simulink model "kopter_se_zavazim_LQR"  (R2024b)
settings: Solver=FixedStepAuto  StartTime=0.0  StopTime=30  FixedStep=0.01  RelTol=1e-3
values from neighbouring files (symbols this model uses):
  b_moment = 5.4e-6    (= 5.4e-06)    [parametry_kopter_se_zavazim.m]
  d = 1    [parametry_kopter_se_zavazim.m]
  g = 9.81    [parametry_kopter_se_zavazim.m]
  Ip = m*d^2    (= 1)    [parametry_kopter_se_zavazim.m]
  Ixx = 0.0222    [parametry_kopter_se_zavazim.m]
  Iyy = 0.0222    [parametry_kopter_se_zavazim.m]
  Izz = 0.0429    [parametry_kopter_se_zavazim.m]
  k_thrust = 2.3e-3    (= 0.0023)    [parametry_kopter_se_zavazim.m]
  ki_lqr = K_ex_lqr(:, 17:20)    [odvozeni_stavova_regulace_OTHER_ANGLES.m]
  kimot_lqr = Kmot_ex_lqr(:, 17:20)    [odvozeni_stavova_regulace_OTHER_ANGLES.m]
  kp_lqr = K_ex_lqr(:, 1:16)    [odvozeni_stavova_regulace_OTHER_ANGLES.m]
  kpmot_lqr = Kmot_ex_lqr(:, 1:16)    [odvozeni_stavova_regulace_OTHER_ANGLES.m]
  l = 0.2051    [parametry_kopter_se_zavazim.m]
  L_observer = place(Ac', Cc', poles_obs)'    [odvozeni_stavova_regulace_OTHER_ANGLES.m]
  M = 2    [parametry_kopter_se_zavazim.m]
  m = 1    [parametry_kopter_se_zavazim.m]
  Us_p = [(M+m)*g; 0; 0; 0]    [parametry_kopter_se_zavazim.m]
  Xinit_ss = [Xinit_matrix; [0 0 0 0 0 0 0 0]']    [parametry_kopter_se_zavazim.m]
  Xs_p = [0;0;0; 0;0;0; 0;0; 0;0;0; 0;0;0; 0;0]    [parametry_kopter_se_zavazim.m]
undefined symbols (not defined in the file or in its folder): L
libraries: simulink_extras x10
(part 1 of 3)
settings Model: Creator=Admin  LastModifiedBy=Admin

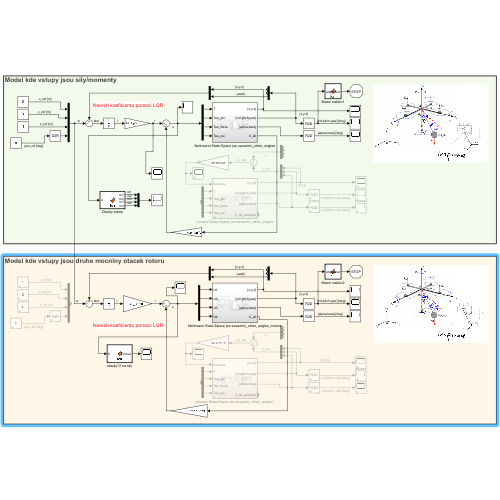
[thumbnail: Simulink's stored preview of the top-level diagram]
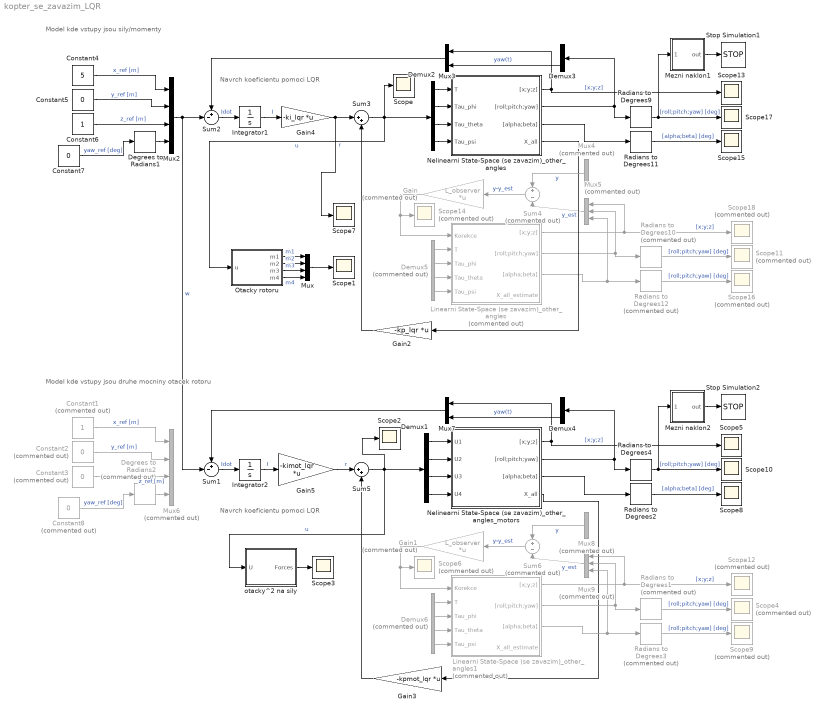
== system kopter_se_zavazim_LQR ==
  note: Navrch koeficientu pomoci LQR
  note: Model kde vstupy jsou sily/momenty
  note: Model kde vstupy jsou druhe mocniny otacek rotoru
  note: Navrch koeficientu pomoci LQR
  Constant1 : Constant  Commented=on
  Constant2 : Constant  Commented=on  Value=0
  Constant3 : Constant  Commented=on  Value=0
  Constant4 : Constant  Value=5
  Constant5 : Constant  Value=0
  Constant6 : Constant
  Constant7 : Constant  Value=0
  Constant8 : Constant  Commented=on  Value=0
  Degrees to Radians1 : simulink_extras/Transformations/Degrees to Radians
  Degrees to Radians2 : simulink_extras/Transformations/Degrees to Radians  Commented=on
  Demux1 : Demux
  Demux2 : Demux
  Demux3 : Demux  Outputs=3
  Demux4 : Demux  Outputs=3
  Demux5 : Demux  Commented=on
  Demux6 : Demux  Commented=on
  Gain : Gain  Commented=on  Gain=L_observer  Multiplication=Matrix(K*u)
  Gain1 : Gain  Commented=on  Gain=L_observer  Multiplication=Matrix(K*u)
  Gain2 : Gain  Gain=-kp_lqr  Multiplication=Matrix(K*u)
  Gain3 : Gain  Gain=-kpmot_lqr  Multiplication=Matrix(K*u)
  Gain4 : Gain  Gain=-ki_lqr  Multiplication=Matrix(K*u)
  Gain5 : Gain  Gain=-kimot_lqr  Multiplication=Matrix(K*u)
  Integrator1 : Integrator
  Integrator2 : Integrator
  Linearni State-Space (se zavazim)_other_angles : Subsystem  Commented=on
  Linearni State-Space (se zavazim)_other_angles1 : Subsystem  Commented=on
  Mezni naklon1 : MATLAB Function  TreatAsAtomicUnit=on
  Mezni naklon2 : MATLAB Function  TreatAsAtomicUnit=on
  Mux : Mux
  Mux2 : Mux
  Mux3 : Mux  Inputs=2
  Mux{4..5,8..9} (4 alike) : Mux  Commented=on  Inputs=3
  Mux6 : Mux  Commented=on
  Mux7 : Mux  Inputs=2
  Nelinearni State-Space (se zavazim)_other_angles : Subsystem
  Nelinearni State-Space (se zavazim)_other_angles_motors : Subsystem
  Otacky rotoru : MATLAB Function  TreatAsAtomicUnit=on
  Radians to Degrees{1,3,10,12} (4 alike) : simulink_extras/Transformations/Radians to Degrees  Commented=on
  Radians to Degrees{2,4,9,11} (4 alike) : simulink_extras/Transformations/Radians to Degrees
  Scope{,1..3,5,7..8,10,13,15,17} (11 alike) : Scope
  Scope{4,6,9,11..12,14,16,18} (8 alike) : Scope  Commented=on
  Stop Simulation1 : Stop
  Stop Simulation2 : Stop
  Sum1 : Sum  Inputs=+-|
  Sum2 : Sum  Inputs=+-|
  Sum3 : Sum  Inputs=|++
  Sum4 : Sum  Commented=on  Inputs=+|-
  Sum5 : Sum  Inputs=|++
  Sum6 : Sum  Commented=on  Inputs=+|-
  otacky^2 na sily : MATLAB Function  TreatAsAtomicUnit=on
  wires:
  Linearni State-Space (se zavazim)_other_angles/1("[x;y;z]") -> Mux5/1, Scope18/1  "[x;y;z]"
  Demux5/3 -> Linearni State-Space (se zavazim)_other_angles/4(Tau_theta)
  Demux5/2 -> Linearni State-Space (se zavazim)_other_angles/3(Tau_phi)
  Nelinearni State-Space (se zavazim)_other_angles/3("[alpha;beta]") -> Radians to Degrees11/1
  Linearni State-Space (se zavazim)_other_angles/3("[alpha;beta]") -> Mux5/3, Radians to Degrees12/1
  Radians to Degrees10/1 -> Scope11/1  "[roll;pitch;yaw] [deg]"
  Linearni State-Space (se zavazim)_other_angles/2("[roll;pitch;yaw]") -> Mux5/2, Radians to Degrees10/1
  Radians to Degrees12/1 -> Scope16/1  "[roll;pitch;yaw] [deg]"
  Demux5/1 -> Linearni State-Space (se zavazim)_other_angles/2(T)
  Demux5/4 -> Linearni State-Space (se zavazim)_other_angles/5(Tau_psi)
  Radians to Degrees9/1 -> Scope17/1, Mezni naklon1/1(angles)  "[roll;pitch;yaw] [deg]"
  Radians to Degrees11/1 -> Scope15/1  "[alpha;beta] [deg]"
  Demux2/3 -> Nelinearni State-Space (se zavazim)_other_angles/3(Tau_theta)
  Demux2/2 -> Nelinearni State-Space (se zavazim)_other_angles/2(Tau_phi)
  Constant5/1 -> Mux2/2  "y_ref [m]"
  Constant7/1 -> Degrees to Radians1/1  "yaw_ref [deg]"
  Constant6/1 -> Mux2/3  "z_ref [m]"
  Gain2/1 -> Sum3/2
  Sum3/1 -> Otacky rotoru/1(u), Scope/1, Demux2/1  "u"
  Mux3/1 -> Sum2/1
  Demux2/4 -> Nelinearni State-Space (se zavazim)_other_angles/4(Tau_psi)
  Sum2/1 -> Integrator1/1  "Idot"
  Gain4/1 -> Scope7/1, Sum3/1  "r"
  Demux2/1 -> Nelinearni State-Space (se zavazim)_other_angles/1(T)
  Integrator1/1 -> Gain4/1  "I"
  Degrees to Radians1/1 -> Mux2/4
  Constant4/1 -> Mux2/1  "x_ref [m]"
  Demux3/3 -> Mux3/2  "yaw(t)"
  Nelinearni State-Space (se zavazim)_other_angles/1("[x;y;z]") -> Scope13/1, Mux3/1  "[x;y;z]"
  Nelinearni State-Space (se zavazim)_other_angles/2("[roll;pitch;yaw]") -> Radians to Degrees9/1, Demux3/1
  Mezni naklon1/1(out) -> Stop Simulation1/1
  Nelinearni State-Space (se zavazim)_other_angles/4(X_all) -> Gain2/1
  Gain/1 -> Scope14/1, Linearni State-Space (se zavazim)_other_angles/1(Korekce)
  Sum4/1 -> Gain/1  "y-y_est"
  Mux4/1 -> Sum4/1  "y"
  Mux5/1 -> Sum4/2  "y_est"
  Otacky rotoru/1(m1) -> Mux/1  "m1"
  Otacky rotoru/2(m2) -> Mux/2  "m2"
  Otacky rotoru/3(m3) -> Mux/3  "m3"
  Otacky rotoru/4(m4) -> Mux/4  "m4"
  Mux/1 -> Scope1/1
  Radians to Degrees4/1 -> Scope10/1, Mezni naklon2/1(angles)  "[roll;pitch;yaw] [deg]"
  Demux6/2 -> Linearni State-Space (se zavazim)_other_angles1/3(Tau_phi)
  Integrator2/1 -> Gain5/1  "I"
  Radians to Degrees2/1 -> Scope8/1  "[alpha;beta] [deg]"
  Gain1/1 -> Scope6/1, Linearni State-Space (se zavazim)_other_angles1/1(Korekce)
  Nelinearni State-Space (se zavazim)_other_angles_motors/4(X_all) -> Gain3/1
  Nelinearni State-Space (se zavazim)_other_angles_motors/2("[roll;pitch;yaw]") -> Radians to Degrees4/1, Demux4/1
  Sum5/1 -> otacky^2 na sily/1(U), Scope2/1, Demux1/1  "u"
  Sum1/1 -> Integrator2/1  "Idot"
  Demux1/2 -> Nelinearni State-Space (se zavazim)_other_angles_motors/2(U2)
  Linearni State-Space (se zavazim)_other_angles1/3("[alpha;beta]") -> Mux9/3, Radians to Degrees3/1
  Degrees to Radians2/1 -> Mux6/4
  Demux6/3 -> Linearni State-Space (se zavazim)_other_angles1/4(Tau_theta)
  Constant2/1 -> Mux6/2  "y_ref [m]"
  Demux4/3 -> Mux7/2  "yaw(t)"
  Demux1/3 -> Nelinearni State-Space (se zavazim)_other_angles_motors/3(U3)
  Constant3/1 -> Mux6/3  "z_ref [m]"
  Mux2/1 -> Sum2/2, Sum1/2  "w"
  Nelinearni State-Space (se zavazim)_other_angles_motors/3("[alpha;beta]") -> Radians to Degrees2/1
  Mux9/1 -> Sum6/2  "y_est"
  Nelinearni State-Space (se zavazim)_other_angles_motors/1("[x;y;z]") -> Scope5/1, Mux7/1  "[x;y;z]"
  Sum6/1 -> Gain1/1  "y-y_est"
  Demux1/1 -> Nelinearni State-Space (se zavazim)_other_angles_motors/1(U1)
  Linearni State-Space (se zavazim)_other_angles1/1("[x;y;z]") -> Mux9/1, Scope12/1  "[x;y;z]"
  Mux7/1 -> Sum1/1
  Mezni naklon2/1(out) -> Stop Simulation2/1
  Radians to Degrees1/1 -> Scope4/1  "[roll;pitch;yaw] [deg]"
  Mux8/1 -> Sum6/1  "y"
  Gain3/1 -> Sum5/2
  Radians to Degrees3/1 -> Scope9/1  "[roll;pitch;yaw] [deg]"
  Gain5/1 -> Sum5/1  "r"
  Linearni State-Space (se zavazim)_other_angles1/2("[roll;pitch;yaw]") -> Mux9/2, Radians to Degrees1/1
  Demux6/1 -> Linearni State-Space (se zavazim)_other_angles1/2(T)
  Demux6/4 -> Linearni State-Space (se zavazim)_other_angles1/5(Tau_psi)
  Demux1/4 -> Nelinearni State-Space (se zavazim)_other_angles_motors/4(U4)
  Constant8/1 -> Degrees to Radians2/1  "yaw_ref [deg]"
  Constant1/1 -> Mux6/1  "x_ref [m]"
  otacky^2 na sily/1(Forces) -> Scope3/1

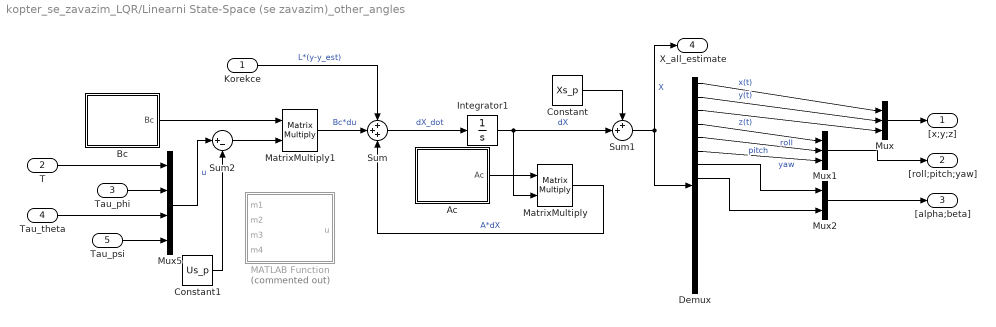
== system kopter_se_zavazim_LQR/Linearni State-Space (se zavazim)_other_angles ==
  Korekce : Inport
  T : Inport  Port=2
  Tau_phi : Inport  Port=3
  Tau_theta : Inport  Port=4
  Tau_psi : Inport  Port=5
  Ac : MATLAB Function  TreatAsAtomicUnit=on
  Bc : MATLAB Function  TreatAsAtomicUnit=on
  Constant : Constant  Value=Xs_p
  Constant1 : Constant  Value=Us_p
  Demux : Demux  Outputs=16
  Integrator1 : Integrator  InitialCondition=Xinit_ss
  MATLAB Function : MATLAB Function  Commented=on  TreatAsAtomicUnit=on
  MatrixMultiply : Product  Multiplication=Matrix(*)
  MatrixMultiply1 : Product  Multiplication=Matrix(*)
  Mux : Mux  Inputs=3
  Mux1 : Mux  Inputs=3
  Mux2 : Mux  Inputs=2
  Mux5 : Mux
  Sum : Sum  Inputs=+++
  Sum1 : Sum  Inputs=++|
  Sum2 : Sum  Inputs=|+-
  "[x;y;z]" : Outport
  "[roll;pitch;yaw]" : Outport  Port=2
  "[alpha;beta]" : Outport  Port=3
  X_all_estimate : Outport  Port=4
  wires:
  Mux5/1 -> Sum2/1  "u"
  Ac/1(Ac) -> MatrixMultiply/1
  Integrator1/1 -> Sum1/2, MatrixMultiply/2  "dX"
  Demux/1 -> Mux/1  "x(t)"
  Demux/2 -> Mux/2  "y(t)"
  Demux/3 -> Mux/3  "z(t)"
  Mux/1 -> "[x;y;z]"/1
  Demux/4 -> Mux1/1  "roll"
  Demux/5 -> Mux1/2  "pitch"
  Demux/6 -> Mux1/3  "yaw"
  Mux1/1 -> "[roll;pitch;yaw]"/1
  Sum/1 -> Integrator1/1  "dX_dot"
  MatrixMultiply1/1 -> Sum/2  "Bc*du"
  MatrixMultiply/1 -> Sum/3  "A*dX"
  Bc/1(Bc) -> MatrixMultiply1/1
  Sum1/1 -> Demux/1, X_all_estimate/1  "X"
  Constant/1 -> Sum1/1
  Constant1/1 -> Sum2/2
  Sum2/1 -> MatrixMultiply1/2
  Mux2/1 -> "[alpha;beta]"/1
  Demux/7 -> Mux2/1
  Demux/8 -> Mux2/2
  Tau_psi/1 -> Mux5/4
  T/1 -> Mux5/1
  Tau_theta/1 -> Mux5/3
  Tau_phi/1 -> Mux5/2
  Korekce/1 -> Sum/1  "L*(y-y_est)"

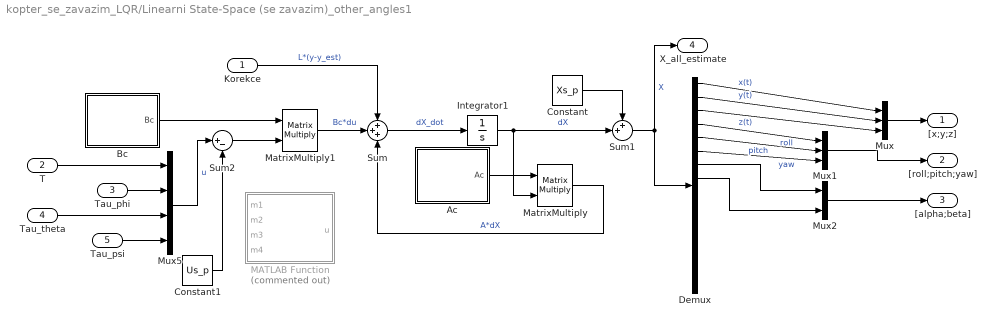
== system kopter_se_zavazim_LQR/Linearni State-Space (se zavazim)_other_angles1 ==
  Korekce : Inport
  T : Inport  Port=2
  Tau_phi : Inport  Port=3
  Tau_theta : Inport  Port=4
  Tau_psi : Inport  Port=5
  Ac : MATLAB Function  TreatAsAtomicUnit=on
  Bc : MATLAB Function  TreatAsAtomicUnit=on
  Constant : Constant  Value=Xs_p
  Constant1 : Constant  Value=Us_p
  Demux : Demux  Outputs=16
  Integrator1 : Integrator  InitialCondition=Xinit_ss
  MATLAB Function : MATLAB Function  Commented=on  TreatAsAtomicUnit=on
  MatrixMultiply : Product  Multiplication=Matrix(*)
  MatrixMultiply1 : Product  Multiplication=Matrix(*)
  Mux : Mux  Inputs=3
  Mux1 : Mux  Inputs=3
  Mux2 : Mux  Inputs=2
  Mux5 : Mux
  Sum : Sum  Inputs=+++
  Sum1 : Sum  Inputs=++|
  Sum2 : Sum  Inputs=|+-
  "[x;y;z]" : Outport
  "[roll;pitch;yaw]" : Outport  Port=2
  "[alpha;beta]" : Outport  Port=3
  X_all_estimate : Outport  Port=4
  wires:
  Mux5/1 -> Sum2/1  "u"
  Ac/1(Ac) -> MatrixMultiply/1
  Integrator1/1 -> Sum1/2, MatrixMultiply/2  "dX"
  Demux/1 -> Mux/1  "x(t)"
  Demux/2 -> Mux/2  "y(t)"
  Demux/3 -> Mux/3  "z(t)"
  Mux/1 -> "[x;y;z]"/1
  Demux/4 -> Mux1/1  "roll"
  Demux/5 -> Mux1/2  "pitch"
  Demux/6 -> Mux1/3  "yaw"
  Mux1/1 -> "[roll;pitch;yaw]"/1
  Sum/1 -> Integrator1/1  "dX_dot"
  MatrixMultiply1/1 -> Sum/2  "Bc*du"
  MatrixMultiply/1 -> Sum/3  "A*dX"
  Bc/1(Bc) -> MatrixMultiply1/1
  Sum1/1 -> Demux/1, X_all_estimate/1  "X"
  Constant/1 -> Sum1/1
  Constant1/1 -> Sum2/2
  Sum2/1 -> MatrixMultiply1/2
  Mux2/1 -> "[alpha;beta]"/1
  Demux/7 -> Mux2/1
  Demux/8 -> Mux2/2
  Tau_psi/1 -> Mux5/4
  T/1 -> Mux5/1
  Tau_theta/1 -> Mux5/3
  Tau_phi/1 -> Mux5/2
  Korekce/1 -> Sum/1  "L*(y-y_est)"

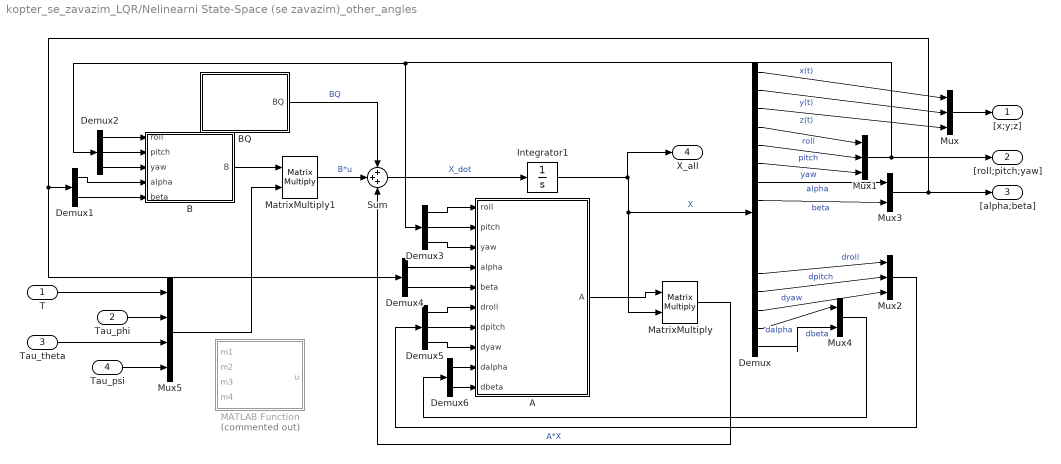
== system kopter_se_zavazim_LQR/Nelinearni State-Space (se zavazim)_other_angles ==
  T : Inport
  Tau_phi : Inport  Port=2
  Tau_theta : Inport  Port=3
  Tau_psi : Inport  Port=4
  A : MATLAB Function  TreatAsAtomicUnit=on
  B : MATLAB Function  TreatAsAtomicUnit=on
  BQ : MATLAB Function  TreatAsAtomicUnit=on
  Demux : Demux  Outputs=16
  Demux1 : Demux  Outputs=2
  Demux2 : Demux  Outputs=3
  Demux3 : Demux  Outputs=3
  Demux4 : Demux  Outputs=2
  Demux5 : Demux  Outputs=3
  Demux6 : Demux  Outputs=2
  Integrator1 : Integrator  InitialCondition=Xinit_ss
  MATLAB Function : MATLAB Function  Commented=on  TreatAsAtomicUnit=on
  MatrixMultiply : Product  Multiplication=Matrix(*)
  MatrixMultiply1 : Product  Multiplication=Matrix(*)
  Mux : Mux  Inputs=3
  Mux1 : Mux  Inputs=3
  Mux2 : Mux  Inputs=3
  Mux3 : Mux  Inputs=2
  Mux4 : Mux  Inputs=2
  Mux5 : Mux
  Sum : Sum  Inputs=+++
  "[x;y;z]" : Outport
  "[roll;pitch;yaw]" : Outport  Port=2
  "[alpha;beta]" : Outport  Port=3
  X_all : Outport  Port=4
  wires:
  A/1(A) -> MatrixMultiply/1
  Integrator1/1 -> X_all/1, MatrixMultiply/2, Demux/1  "X"
  Demux/1 -> Mux/1  "x(t)"
  Demux/2 -> Mux/2  "y(t)"
  Demux/3 -> Mux/3  "z(t)"
  Mux/1 -> "[x;y;z]"/1
  Demux/4 -> Mux1/1  "roll"
  Demux/5 -> Mux1/2  "pitch"
  Demux/6 -> Mux1/3  "yaw"
  Mux1/1 -> Demux2/1, Demux3/1, "[roll;pitch;yaw]"/1
  Demux/12 -> Mux2/1  "droll"
  Demux/13 -> Mux2/2  "dpitch"
  Demux/14 -> Mux2/3  "dyaw"
  Demux2/1 -> B/1(roll)
  Demux2/2 -> B/2(pitch)
  Demux2/3 -> B/3(yaw)
  Demux3/2 -> A/2(pitch)
  Demux3/1 -> A/1(roll)
  Demux3/3 -> A/3(yaw)
  Demux5/2 -> A/7(dpitch)
  Demux5/1 -> A/6(droll)
  Demux5/3 -> A/8(dyaw)
  Sum/1 -> Integrator1/1  "X_dot"
  BQ/1(BQ) -> Sum/1  "BQ"
  MatrixMultiply1/1 -> Sum/2  "B*u"
  B/1(B) -> MatrixMultiply1/1
  MatrixMultiply/1 -> Sum/3  "A*X"
  Mux2/1 -> Demux5/1
  Demux/7 -> Mux3/1  "alpha"
  Demux/8 -> Mux3/2  "beta"
  Mux3/1 -> Demux4/1, Demux1/1, "[alpha;beta]"/1
  Demux1/2 -> B/5(beta)
  Demux1/1 -> B/4(alpha)
  Demux4/2 -> A/5(beta)
  Demux4/1 -> A/4(alpha)
  Demux/15 -> Mux4/1  "dalpha"
  Demux/16 -> Mux4/2  "dbeta"
  Demux6/1 -> A/9(dalpha)
  Demux6/2 -> A/10(dbeta)
  Mux4/1 -> Demux6/1
  Tau_theta/1 -> Mux5/3
  Tau_psi/1 -> Mux5/4
  Tau_phi/1 -> Mux5/2
  Mux5/1 -> MatrixMultiply1/2
  T/1 -> Mux5/1

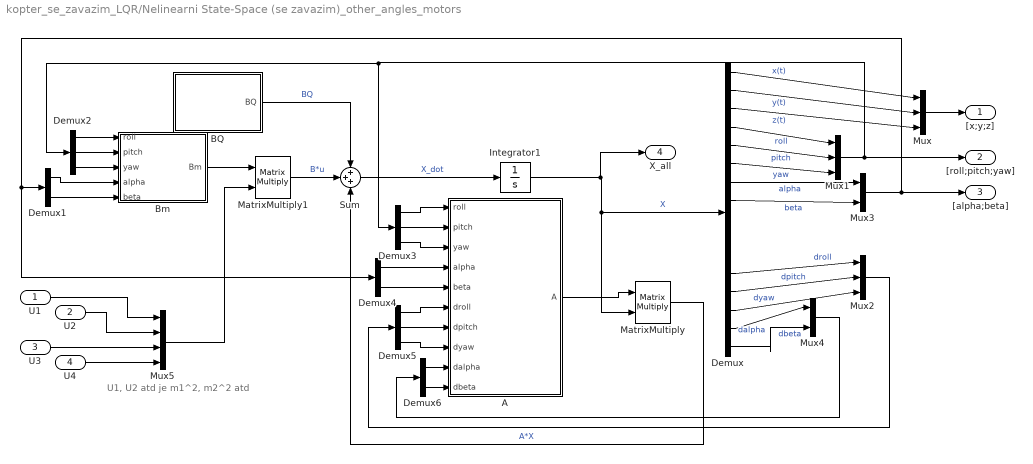
== system kopter_se_zavazim_LQR/Nelinearni State-Space (se zavazim)_other_angles_motors ==
  note: U1, U2 atd je m1^2, m2^2 atd
  U1 : Inport
  U2 : Inport  Port=2
  U3 : Inport  Port=3
  U4 : Inport  Port=4
  A : MATLAB Function  TreatAsAtomicUnit=on
  BQ : MATLAB Function  TreatAsAtomicUnit=on
  Bm : MATLAB Function  TreatAsAtomicUnit=on
  Demux : Demux  Outputs=16
  Demux1 : Demux  Outputs=2
  Demux2 : Demux  Outputs=3
  Demux3 : Demux  Outputs=3
  Demux4 : Demux  Outputs=2
  Demux5 : Demux  Outputs=3
  Demux6 : Demux  Outputs=2
  Integrator1 : Integrator  InitialCondition=Xinit_ss
  MatrixMultiply : Product  Multiplication=Matrix(*)
  MatrixMultiply1 : Product  Multiplication=Matrix(*)
  Mux : Mux  Inputs=3
  Mux1 : Mux  Inputs=3
  Mux2 : Mux  Inputs=3
  Mux3 : Mux  Inputs=2
  Mux4 : Mux  Inputs=2
  Mux5 : Mux
  Sum : Sum  Inputs=+++
  "[x;y;z]" : Outport
  "[roll;pitch;yaw]" : Outport  Port=2
  "[alpha;beta]" : Outport  Port=3
  X_all : Outport  Port=4
  wires:
  A/1(A) -> MatrixMultiply/1
  Integrator1/1 -> X_all/1, MatrixMultiply/2, Demux/1  "X"
  Demux/1 -> Mux/1  "x(t)"
  Demux/2 -> Mux/2  "y(t)"
  Demux/3 -> Mux/3  "z(t)"
  Mux/1 -> "[x;y;z]"/1
  Demux/4 -> Mux1/1  "roll"
  Demux/5 -> Mux1/2  "pitch"
  Demux/6 -> Mux1/3  "yaw"
  Mux1/1 -> Demux2/1, Demux3/1, "[roll;pitch;yaw]"/1
  Demux/12 -> Mux2/1  "droll"
  Demux/13 -> Mux2/2  "dpitch"
  Demux/14 -> Mux2/3  "dyaw"
  Demux2/1 -> Bm/1(roll)
  Demux2/2 -> Bm/2(pitch)
  Demux2/3 -> Bm/3(yaw)
  Demux3/2 -> A/2(pitch)
  Demux3/1 -> A/1(roll)
  Demux3/3 -> A/3(yaw)
  Demux5/2 -> A/7(dpitch)
  Demux5/1 -> A/6(droll)
  Demux5/3 -> A/8(dyaw)
  Sum/1 -> Integrator1/1  "X_dot"
  BQ/1(BQ) -> Sum/1  "BQ"
  MatrixMultiply1/1 -> Sum/2  "B*u"
  Bm/1(Bm) -> MatrixMultiply1/1
  MatrixMultiply/1 -> Sum/3  "A*X"
  Mux2/1 -> Demux5/1
  Demux/7 -> Mux3/1  "alpha"
  Demux/8 -> Mux3/2  "beta"
  Mux3/1 -> Demux4/1, Demux1/1, "[alpha;beta]"/1
  Demux1/2 -> Bm/5(beta)
  Demux1/1 -> Bm/4(alpha)
  Demux4/2 -> A/5(beta)
  Demux4/1 -> A/4(alpha)
  Demux/15 -> Mux4/1  "dalpha"
  Demux/16 -> Mux4/2  "dbeta"
  Demux6/1 -> A/9(dalpha)
  Demux6/2 -> A/10(dbeta)
  Mux4/1 -> Demux6/1
  Mux5/1 -> MatrixMultiply1/2
  U4/1 -> Mux5/4
  U3/1 -> Mux5/3
  U2/1 -> Mux5/2
  U1/1 -> Mux5/1

== matlab function kopter_se_zavazim_LQR/Linearni State-Space (se zavazim)_other_angles1/MATLAB Function ==
  data: u output; m1 input; m2 input; m3 input; m4 input; k_thrust parameter; b_moment parameter; L parameter
function u = fcn(m1, m2, m3, m4, k_thrust, b_moment, L)

Thrust = k_thrust*(m1^2 + m2^2 + m3^2 + m4^2);
Tau_roll = L*k_thrust*(m1^2 + m4^2 - m2^2 - m3^2);
Tau_pitch = L*k_thrust*(m4^2 + m3^2 - m1^2 - m2^2);
Tau_yaw = b_moment*(m1^2 + m3^2 - m2^2 - m4^2);

u = [Thrust; Tau_roll; Tau_pitch; Tau_yaw];

== matlab function kopter_se_zavazim_LQR/Mezni naklon2 ==
  data: angles input; out output
function out = fcn(angles)

if all(angles<=85) && all(angles>=-85)
    out = 0;
else
    out = 1;
end

== matlab function kopter_se_zavazim_LQR/Nelinearni State-Space (se zavazim)_other_angles_motors/A ==
  data: roll input; A output; pitch input; yaw input; alpha input; beta input; droll input; dpitch input; dyaw input; dalpha input; dbeta input; Ixx parameter; Iyy parameter; Izz parameter; M parameter; Ip parameter; d parameter; m parameter
function A = fcn(roll, pitch, yaw, alpha, beta, droll, dpitch, dyaw, dalpha, dbeta, Ixx, Iyy, Izz, M, Ip, d, m)
% Matice dynamiky A

phi_t = roll;
theta_t = pitch;
psi_t = yaw;

alpha_t = alpha;
beta_t = beta;

phi_dot_t = droll;
theta_dot_t = dpitch;
psi_dot_t = dyaw;

alpha_dot_t = dalpha;
beta_dot_t = dbeta;

A = [ 
0, 0, 0, 0, 0, 0, 0, 0, 1, 0, 0,                                                                                                                                                                                                                                                                                                                                                                                                                                                                                                           0,                                                                                                                                                                                                                                                                                                                                                                                                                                                                                                                                                                                                                                                                                                                              0,                                                                                                                                                                                            0,                                                          0,                                                  0;
0, 0, 0, 0, 0, 0, 0, 0, 0, 1, 0,                                                                                                                                                                                                                                                                                                                                                                                                                                                                                                           0,                                                                                                                                                                                                                                                                                                                                                                                                                                                                                                                                                                                                                                                                                                                              0,                                                                                                                                                                                            0,                                                          0,                                                  0;
0, 0, 0, 0, 0, 0, 0, 0, 0, 0, 1,                                                                                                                                                                                                                                                                                                                                                                                                                                                                                                           0,                                                                                                                                                                                                                                                                                                                                                                                                                                                                                                                                                                                                                                                                                                                              0,                                                                                                                                                                                            0,                                                          0,                                                  0;
0, 0, 0, 0, 0, 0, 0, 0, 0, 0, 0,                                                                                                                                                                                                                                                                                                                                                                                                                                                                                                           1,                                                                                                                                                                                                                                                                                                                                                                                                                                                                                                                                                                                                                                                                                                                              0,                                                                                                                                                                                            0,                                                          0,                                                  0;
0, 0, 0, 0, 0, 0, 0, 0, 0, 0, 0,                                                                                                                                                                                                                                                                                                                                                                                                                                                                                                           0,                                                                                                                                                                                                                                                                                                                                                                                                                                                                                                                                                                                                                                                                                                                              1,                                                                                                                                                                                            0,                                                          0,                                                  0;
0, 0, 0, 0, 0, 0, 0, 0, 0, 0, 0,                                                                                                                                                                                                                                                                                                                                                                                                                                                                                                           0,                                                                                                                                                                                                                                                                                                                                                                                                                                                                                                                                                                                                                                                                                                                              0,                                                                                                                                                                                            1,                                                          0,                                                  0;
0, 0, 0, 0, 0, 0, 0, 0, 0, 0, 0,                                                                                                                                                                                                                                                                                                                                                                                                                                                                                                           0,                                                                                                                                                                                                                                                                                                                                                                                                                                                                                                                                                                                                                                                                                                                              0,                                                                                                                                                                                            0,                                                          1,                                                  0;
0, 0, 0, 0, 0, 0, 0, 0, 0, 0, 0,                                                                                                                                                                                                                                                                                                                                                                                                                                                                                                           0,                                                                                                                                                                                                                                                                                                                                                                                                                                                                                                                                                                                                                                                                                                                              0,                                                                                                                                                                                            0,                                                          0,                                                  1;
0, 0, 0, 0, 0, 0, 0, 0, 0, 0, 0,                                                                                                                                                                                                                                                                                                                                                                                                                                                                                                           0,                                                                                                                                                                                                                                                                                                                                                                                                                                                                                                                                                                                                                                                                                                                              0,                                                                                                                                                                                            0,       (alpha_dot_t*d*m*cos(beta_t)^3*sin(alpha_t))/(M + m),  (beta_dot_t*d*m*cos(beta_t)*sin(alpha_t))/(M + m);
0, 0, 0, 0, 0, 0, 0, 0, 0, 0, 0,                                                                                                                                                                                                                                                                                                                                                                                                                                                                                                           0,                                                                                                                                                                                                                                                                                                                                                                                                                                                                                                                                                                                                                                                                                                                              0,                                                                                                                                                                                            0, -(alpha_dot_t*d*m*sin(beta_t)*(sin(beta_t)^2 - 1))/(M + m),               (beta_dot_t*d*m*sin(beta_t))/(M + m);
0, 0, 0, 0, 0, 0, 0, 0, 0, 0, 0,                                                                                                                                                                                                                                                                                                                                                                                                                                                                                                           0,                                                                                                                                                                                                                                                                                                                                                                                                                                                                                                                                                                                                                                                                                                                              0,                                                                                                                                                                                            0,      -(alpha_dot_t*d*m*cos(alpha_t)*cos(beta_t)^3)/(M + m), -(beta_dot_t*d*m*cos(alpha_t)*cos(beta_t))/(M + m);
0, 0, 0, 0, 0, 0, 0, 0, 0, 0, 0,                                       (sin(theta_t)*(Ixx*Izz*theta_dot_t - Izz^2*theta_dot_t + Iyy*Izz*theta_dot_t - Iyy^2*theta_dot_t*cos(phi_t)^2 + Izz^2*theta_dot_t*cos(phi_t)^2 + Ixx*Iyy*theta_dot_t*cos(phi_t)^2 - Ixx*Izz*theta_dot_t*cos(phi_t)^2 - Iyy^2*psi_dot_t*cos(phi_t)*cos(theta_t)*sin(phi_t) + Izz^2*psi_dot_t*cos(phi_t)*cos(theta_t)*sin(phi_t) + Ixx*Iyy*psi_dot_t*cos(phi_t)*cos(theta_t)*sin(phi_t) - Ixx*Izz*psi_dot_t*cos(phi_t)*cos(theta_t)*sin(phi_t)))/(Iyy*Izz*cos(theta_t)), - ((Iyy*Izz + Ixx*Iyy*sin(theta_t)^2 - Iyy*Izz*sin(theta_t)^2 - Ixx*Iyy*sin(phi_t)^2*sin(theta_t)^2 + Ixx*Izz*sin(phi_t)^2*sin(theta_t)^2)*((Izz*theta_dot_t*sin(2*phi_t))/2 - (Iyy*theta_dot_t*sin(2*phi_t))/2 + Ixx*psi_dot_t*cos(theta_t) - Iyy*psi_dot_t*cos(theta_t) + Izz*psi_dot_t*cos(theta_t) + 2*Iyy*psi_dot_t*cos(phi_t)^2*cos(theta_t) - 2*Izz*psi_dot_t*cos(phi_t)^2*cos(theta_t)))/(Ixx*Iyy*Izz*(sin(theta_t)^2 - 1)) - (sin(theta_t)^2*(Iyy - Iyy*sin(phi_t)^2 + Izz*sin(phi_t)^2)*((Iyy*theta_dot_t*sin(2*phi_t))/2 - (Izz*theta_dot_t*sin(2*phi_t))/2 - 2*Ixx*psi_dot_t*cos(theta_t) + 2*Izz*psi_dot_t*cos(phi_t)^2*cos(theta_t) + 2*Iyy*psi_dot_t*cos(theta_t)*sin(phi_t)^2))/(Iyy*Izz*(sin(theta_t)^2 - 1)), (psi_dot_t*sin(2*phi_t)*(Iyy - Izz)*(Ixx^2*cos(2*theta_t) - Ixx^2 + Ixx*Iyy + Ixx*Izz + Iyy*Izz - Ixx*Iyy*cos(2*theta_t) - Ixx*Izz*cos(2*theta_t) + Iyy*Izz*cos(2*theta_t)))/(4*Ixx*Iyy*Izz),                                                          0,                                                  0;
0, 0, 0, 0, 0, 0, 0, 0, 0, 0, 0, -(Izz^2*theta_dot_t*sin(2*phi_t) - Izz^2*psi_dot_t*cos(theta_t) - Iyy^2*theta_dot_t*sin(2*phi_t) - Iyy^2*psi_dot_t*cos(theta_t) + Ixx*Iyy*psi_dot_t*cos(theta_t) + Ixx*Izz*psi_dot_t*cos(theta_t) + 2*Iyy*Izz*psi_dot_t*cos(theta_t) + Iyy^2*psi_dot_t*cos(2*phi_t)*cos(theta_t) - Izz^2*psi_dot_t*cos(2*phi_t)*cos(theta_t) + Ixx*Iyy*theta_dot_t*sin(2*phi_t) - Ixx*Izz*theta_dot_t*sin(2*phi_t) - Ixx*Iyy*psi_dot_t*cos(2*phi_t)*cos(theta_t) + Ixx*Izz*psi_dot_t*cos(2*phi_t)*cos(theta_t))/(2*Iyy*Izz),                                                                                                                                                                                                                                                                                                                                                                                                                                                                                                                                                                                                                                        -(psi_dot_t*cos(phi_t)*sin(phi_t)*sin(theta_t)*(Iyy - Izz)*(Iyy - Ixx + Izz))/(Iyy*Izz),                           (psi_dot_t*sin(2*theta_t)*(Iyy^2*cos(2*phi_t) - Izz^2*cos(2*phi_t) - Iyy^2 - Izz^2 + Ixx*Iyy + Ixx*Izz - Ixx*Iyy*cos(2*phi_t) + Ixx*Izz*cos(2*phi_t)))/(4*Iyy*Izz),                                                          0,                                                  0;
0, 0, 0, 0, 0, 0, 0, 0, 0, 0, 0,                                            (Ixx*Iyy*theta_dot_t - Izz^2*theta_dot_t - Iyy^2*theta_dot_t + Ixx*Izz*theta_dot_t + 2*Iyy*Izz*theta_dot_t - Iyy^2*theta_dot_t*cos(2*phi_t) + Izz^2*theta_dot_t*cos(2*phi_t) - Iyy^2*psi_dot_t*sin(2*phi_t)*cos(theta_t) + Izz^2*psi_dot_t*sin(2*phi_t)*cos(theta_t) + Ixx*Iyy*theta_dot_t*cos(2*phi_t) - Ixx*Izz*theta_dot_t*cos(2*phi_t) + Ixx*Iyy*psi_dot_t*sin(2*phi_t)*cos(theta_t) - Ixx*Izz*psi_dot_t*sin(2*phi_t)*cos(theta_t))/(2*Iyy*Izz*cos(theta_t)),                                                                                                                                                                                                                                                                                                                                                                                                                                                                                                                                                                                                                  (psi_dot_t*sin(theta_t)*(Iyy - Iyy*sin(phi_t)^2 + Izz*sin(phi_t)^2)*(Iyy - Ixx + Izz))/(Iyy*Izz*cos(theta_t)),                                                                                                       (psi_dot_t*cos(phi_t)*sin(phi_t)*sin(theta_t)*(Iyy - Izz)*(Iyy - Ixx + Izz))/(Iyy*Izz),                                                          0,                                                  0;
0, 0, 0, 0, 0, 0, 0, 0, 0, 0, 0,                                                                                                                                                                                                                                                                                                                                                                                                                                                                                                           0,                                                                                                                                                                                                                                                                                                                                                                                                                                                                                                                                                                                                                                                                                                                              0,                                                                                                                                                                                            0,                     (2*beta_dot_t*sin(beta_t))/cos(beta_t),                                                  0;
0, 0, 0, 0, 0, 0, 0, 0, 0, 0, 0,                                                                                                                                                                                                                                                                                                                                                                                                                                                                                                           0,                                                                                                                                                                                                                                                                                                                                                                                                                                                                                                                                                                                                                                                                                                                              0,                                                                                                                                                                                            0,                             -(alpha_dot_t*sin(2*beta_t))/2,                                                  0];
